simulink model "EX1"  (R2023a)
settings: Solver=VariableStepAuto  StartTime=0.0  StopTime=5e-4  RelTol=1e-3
values from neighbouring files (symbols this model uses):
  C = 1e-7    (= 1e-07)    [ex1prg1example.m]
  L = 2e-3    (= 0.002)    [ex1prg1example.m]
  R = 100    [ex1prg1example.m]
settings Model: Creator=Roy  LastModifiedBy=Roy

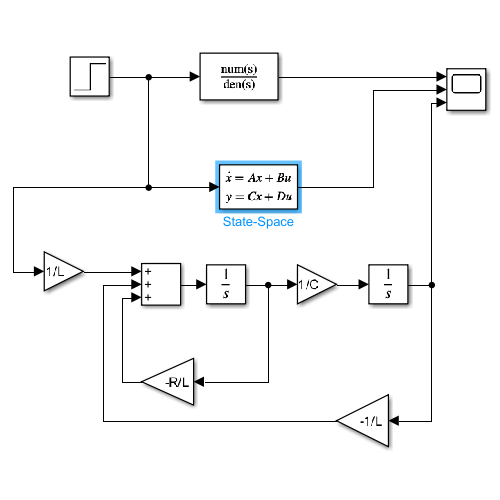
[thumbnail: Simulink's stored preview of the top-level diagram]
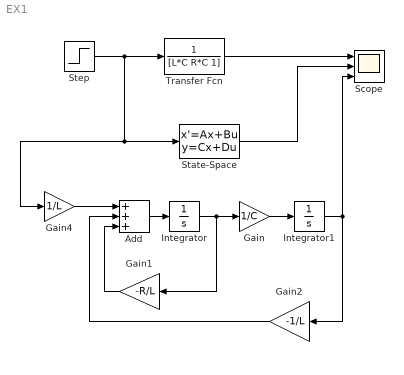
== system EX1 ==
  Add : Sum  Inputs=+++
  Gain : Gain  Gain=1/C
  Gain1 : Gain  Gain=-R/L
  Gain2 : Gain  Gain=-1/L
  Gain4 : Gain  Gain=1/L
  Integrator : Integrator
  Integrator1 : Integrator
  Scope : Scope  NumInputPorts=3
  State-Space : StateSpace  A=[-R/L,-1/L;1/C,0]  B=[1/L;0]  C=[0,1]  D=0  InitialCondition=0
  Step : Step  Time=1e-4  SampleTime=0
  Transfer Fcn : TransferFcn  Denominator=[L*C R*C 1]
  wires:
  Transfer Fcn/1 -> Scope/1
  Step/1 -> Gain4/1, State-Space/1, Transfer Fcn/1
  Add/1 -> Integrator/1
  Integrator/1 -> Gain1/1, Gain/1
  Gain/1 -> Integrator1/1
  Integrator1/1 -> Gain2/1, Scope/3
  Gain1/1 -> Add/3
  Gain4/1 -> Add/1
  Gain2/1 -> Add/2
  State-Space/1 -> Scope/2
